simulink model "lab2q7"  (R2026a)
settings: Solver=ode45  StopTime=1  MaxStep=0.2
libraries: dspfdesign x2, commchan3 x1
settings Model: Creator=steve  LastModifiedBy=steve

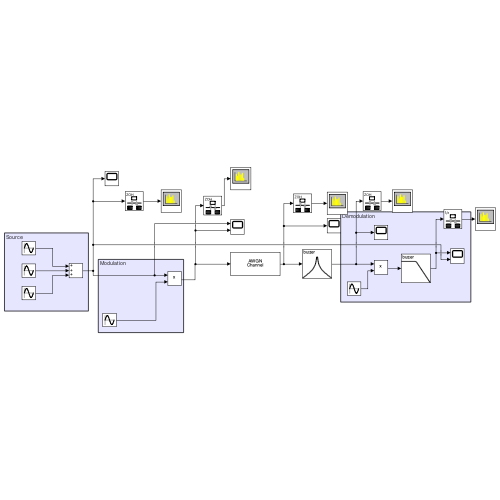
[thumbnail: Simulink's stored preview of the top-level diagram]
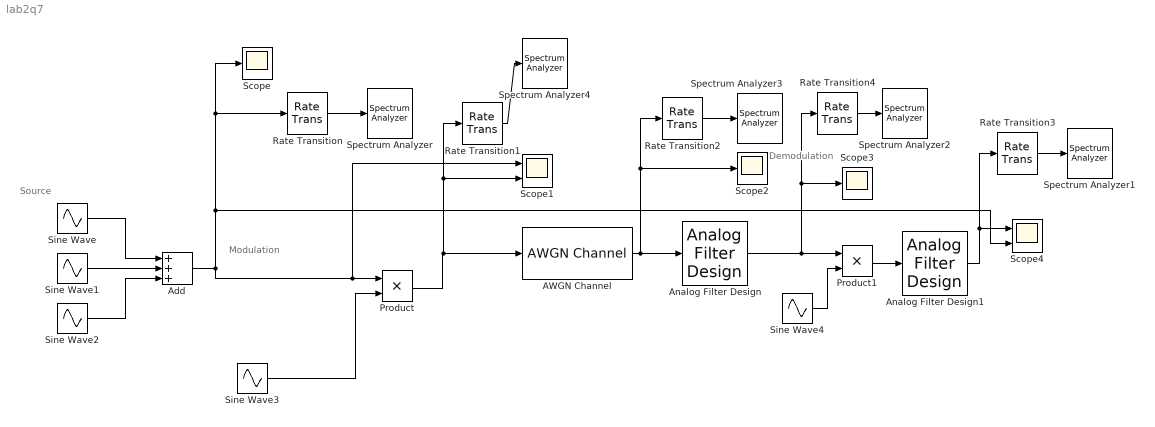
== system lab2q7 ==
  note: Demodulation
  note: Modulation
  note: Source
  AWGN Channel : commchan3/AWGN Channel  LegacyMode=off  NoiseMethod=Variance  noiseMode="Signal to noise ratio  (SNR)"  EbNo=10  EsNo=10  SNR=10  BitsPerSymbol=1  SignalPower=1  SpecifySymbolPeriod=off  SamplesPerSymbol=1  SymbolPeriod=1  VarianceSource=Parameter  Variance=1e-2  RandomStream=mt19937ar with seed  Seed=9876  SimulateUsing=Code generation
  Add : Sum  Inputs=+++
  Analog Filter Design : dspfdesign/Analog Filter Design  method=Butterworth  filttype=Bandpass  N=8  Wlo=14300*2*pi  Whi=15800*2*pi  Rp=2  Rs=40
  Analog Filter Design1 : dspfdesign/Analog Filter Design  method=Butterworth  filttype=Lowpass  N=8  Wlo=800*2*pi  Whi=80  Rp=2  Rs=40
  Product : Product
  Product1 : Product
  Rate Transition{,1..4} (5 alike) : RateTransition  OutPortSampleTime=2e-5
  Scope : Scope
      settings: ActiveDisplayYMinimum=-6.1073523879924263  ActiveDisplayYMaximum=6.1073523950560222
  Scope1 : Scope  NumInputPorts=2
      settings: ActiveDisplayYMinimum=-13.593064225734054  ActiveDisplayYMaximum=13.605764821471759
  Scope2 : Scope
      settings: DataLoggingVariableName=ScopeData2
  Scope3 : Scope
      settings: DataLoggingVariableName=ScopeData3
  Scope4 : Scope  NumInputPorts=2
      settings: ActiveDisplayYMinimum=-6.2949805323797685  ActiveDisplayYMaximum=7.796005675125838  DataLoggingVariableName=ScopeData4
  Sine Wave : Sin  Frequency=1000*pi  SampleTime=0
  Sine Wave1 : Sin  Amplitude=3  Frequency=600*pi  SampleTime=0
  Sine Wave2 : Sin  Amplitude=1.5  Frequency=1200*pi  SampleTime=0
  Sine Wave3 : Sin  Frequency=30000*pi  Phase=pi/2  SampleTime=0
  Sine Wave4 : Sin  Frequency=30000*pi  Phase=pi/2  SampleTime=0
  Spectrum Analyzer : SpectrumAnalyzer  WindowPosition=[1.000000,67.000000,1470.000000,824.000000,]  ScopeFrameLocation=window  RBWSource=Property  RBW=0.5  WindowInvariantSamplesPerUpdate=on  YLimits=[-379.4682 79.4094]  SelectedToolstripTab=spectrumAnalyzerToolstrip.measurementsTab
  Spectrum Analyzer1 : SpectrumAnalyzer  WindowPosition=[1.000000,67.000000,1470.000000,824.000000,]  ScopeFrameLocation=window  RBWSource=Property  RBW=10  WindowInvariantSamplesPerUpdate=on  YLimits=[-74.10680779238224 55.144165967619564]  SelectedToolstripTab=spectrumAnalyzerToolstrip.measurementsTab
  Spectrum Analyzer2 : SpectrumAnalyzer  WindowPosition=[1.000000,67.000000,1470.000000,824.000000,]  ScopeFrameLocation=window  RBWSource=Property  RBW=10  WindowInvariantSamplesPerUpdate=on  YLimits=[-72.1581 38.3902]  SelectedToolstripTab=spectrumAnalyzerToolstrip.measurementsTab
  Spectrum Analyzer3 : SpectrumAnalyzer  WindowPosition=[1.000000,67.000000,1470.000000,824.000000,]  ScopeFrameLocation=window  RBWSource=Property  RBW=10  WindowInvariantSamplesPerUpdate=on  YLimits=[-65.8505 37.8872]  SelectedToolstripTab=spectrumAnalyzerToolstrip.measurementsTab
  Spectrum Analyzer4 : SpectrumAnalyzer  WindowPosition=[1.000000,67.000000,1470.000000,824.000000,]  ScopeFrameLocation=window  RBWSource=Property  RBW=10  WindowInvariantSamplesPerUpdate=on  YLimits=[-285.1798 62.2436]  SelectedToolstripTab=spectrumAnalyzerToolstrip.measurementsTab
  wires:
  Sine Wave/1 -> Add/1
  Sine Wave1/1 -> Add/2
  Sine Wave2/1 -> Add/3
  Rate Transition/1 -> Spectrum Analyzer/1
  Sine Wave3/1 -> Product/2
  Add/1 -> Scope1/1, Product/1, Scope4/2, Scope/1, Rate Transition/1
  Product/1 -> Rate Transition1/1, Scope1/2, AWGN Channel/1
  Rate Transition1/1 -> Spectrum Analyzer4/1
  AWGN Channel/1 -> Scope2/1, Rate Transition2/1, Analog Filter Design/1
  Rate Transition2/1 -> Spectrum Analyzer3/1
  Analog Filter Design/1 -> Product1/1, Scope3/1, Rate Transition4/1
  Rate Transition4/1 -> Spectrum Analyzer2/1
  Rate Transition3/1 -> Spectrum Analyzer1/1
  Sine Wave4/1 -> Product1/2
  Product1/1 -> Analog Filter Design1/1
  Analog Filter Design1/1 -> Rate Transition3/1, Scope4/1
